simulink model "PCM"  (R2018b)
settings: Solver=VariableStepAuto  StartTime=0.0  StopTime=10.0  RelTol=1e-3
libraries: commutil2 x3
settings Model: Creator=Aurora  LastModifiedBy=Aurora

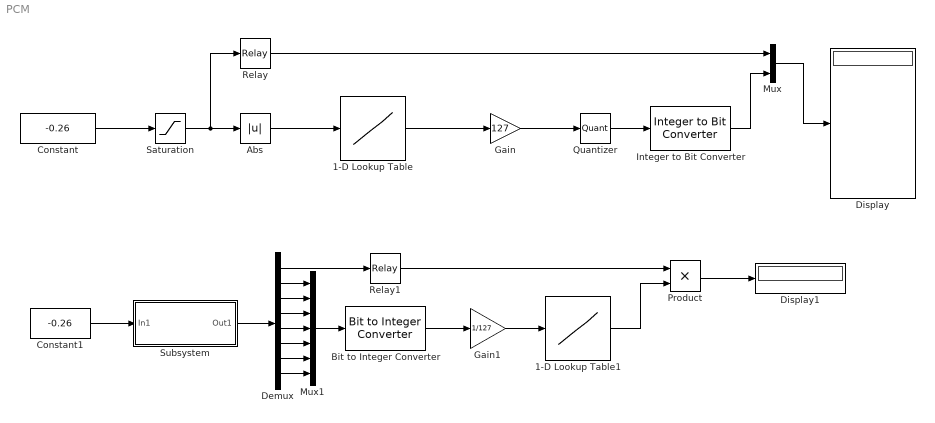
== system PCM ==
  1-D Lookup Table : Lookup_n-D  NumberOfTableDimensions=1  BreakpointsForDimension1=[0,1/128,1/64,1/32,1/16,1/8,1/4,1/2,1]  Table=[0:1/8:1]  InternalRulePriority=Speed  RndMeth=Simplest  InputSameDT=on
  1-D Lookup Table1 : Lookup_n-D  NumberOfTableDimensions=1  BreakpointsForDimension1=[0:1/8:1]  Table=[0,1/128,1/64,1/32,1/16,1/8,1/4,1/2,1]  InternalRulePriority=Speed  RndMeth=Simplest  InputSameDT=on
  Abs : Abs
  Bit to Integer Converter : commutil2/Bit to Integer Converter  nbits=7  bitOrder=MSB first  signedOutputValues=Unsigned  outDtype=Inherit via internal rule  outDtypeSigned=Inherit via internal rule
  Constant : Constant  Value=-0.26
  Constant1 : Constant  Value=-0.26
  Demux : Demux  Outputs=8
  Display : Display
  Display1 : Display
  Gain : Gain  Gain=127
  Gain1 : Gain  Gain=1/127
  Integer to Bit Converter : commutil2/Integer to Bit Converter  nbits=7  signedInputValues=Unsigned  bitOrder=MSB first  outDtype=Inherit via internal rule
  Mux : Mux  Inputs=2
  Mux1 : Mux  Inputs=7
  Product : Product
  Quantizer : Quantizer  QuantizationInterval=1
  Relay : Relay
  Relay1 : Relay  OnSwitchValue=0.5  OffSwitchValue=0.5  OffOutputValue=-1
  Saturation : Saturate  UpperLimit=1  LowerLimit=-1
  Subsystem : Subsystem
  wires:
  Constant/1 -> Saturation/1
  Saturation/1 -> Relay/1, Abs/1
  1-D Lookup Table/1 -> Gain/1
  Gain/1 -> Quantizer/1
  Quantizer/1 -> Integer to Bit Converter/1
  Abs/1 -> 1-D Lookup Table/1
  Relay/1 -> Mux/1
  Integer to Bit Converter/1 -> Mux/2
  Mux/1 -> Display/1
  Relay1/1 -> Product/1
  Demux/5 -> Mux1/4
  Demux/7 -> Mux1/6
  Demux/3 -> Mux1/2
  Mux1/1 -> Bit to Integer Converter/1
  Demux/1 -> Relay1/1
  Constant1/1 -> Subsystem/1(In1)
  Demux/4 -> Mux1/3
  1-D Lookup Table1/1 -> Product/2
  Demux/2 -> Mux1/1
  Demux/6 -> Mux1/5
  Bit to Integer Converter/1 -> Gain1/1
  Subsystem/1(Out1) -> Demux/1
  Product/1 -> Display1/1
  Demux/8 -> Mux1/7
  Gain1/1 -> 1-D Lookup Table1/1

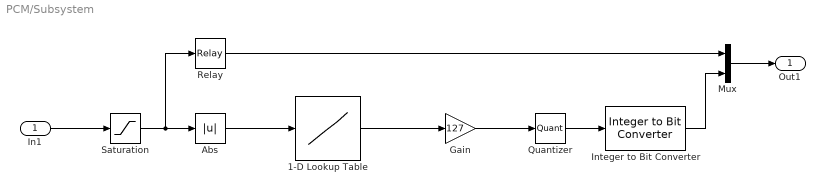
== system PCM/Subsystem ==
  In1 : Inport
  1-D Lookup Table : Lookup_n-D  NumberOfTableDimensions=1  BreakpointsForDimension1=[0,1/128,1/64,1/32,1/16,1/8,1/4,1/2,1]  Table=[0:1/8:1]  InternalRulePriority=Speed  RndMeth=Simplest  InputSameDT=on
  Abs : Abs
  Gain : Gain  Gain=127
  Integer to Bit Converter : commutil2/Integer to Bit Converter  nbits=7  signedInputValues=Unsigned  bitOrder=MSB first  outDtype=Inherit via internal rule
  Mux : Mux  Inputs=2
  Quantizer : Quantizer  QuantizationInterval=1
  Relay : Relay
  Saturation : Saturate  UpperLimit=1  LowerLimit=-1
  Out1 : Outport
  wires:
  Abs/1 -> 1-D Lookup Table/1
  Quantizer/1 -> Integer to Bit Converter/1
  Gain/1 -> Quantizer/1
  1-D Lookup Table/1 -> Gain/1
  In1/1 -> Saturation/1
  Integer to Bit Converter/1 -> Mux/2
  Relay/1 -> Mux/1
  Saturation/1 -> Relay/1, Abs/1
  Mux/1 -> Out1/1
